simulink model "eurofusion_force_control"  (R2025b)
settings: Solver=ode1  StartTime=0.0  StopTime=100  FixedStep=dt  RelTol=1e-3
model workspace (MAT data in the model file):
  Kd_orient_value = 10
  Kd_pos_value = 100
  Kf_pos = 1
  Kf_rot = 1
  Kp_orient_value = 1
  Kp_pos_value = 1
  Md_pos = 1
  Md_rot = 1
  dt = 0.001
libraries: sdu_controllers x5
settings Model: Creator=eld  LastModifiedBy=madla

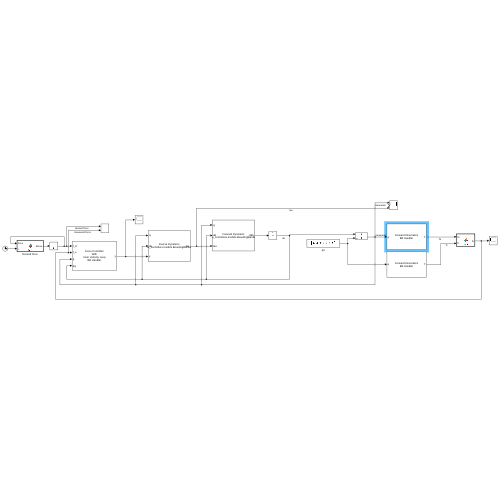
[thumbnail: Simulink's stored preview of the top-level diagram]
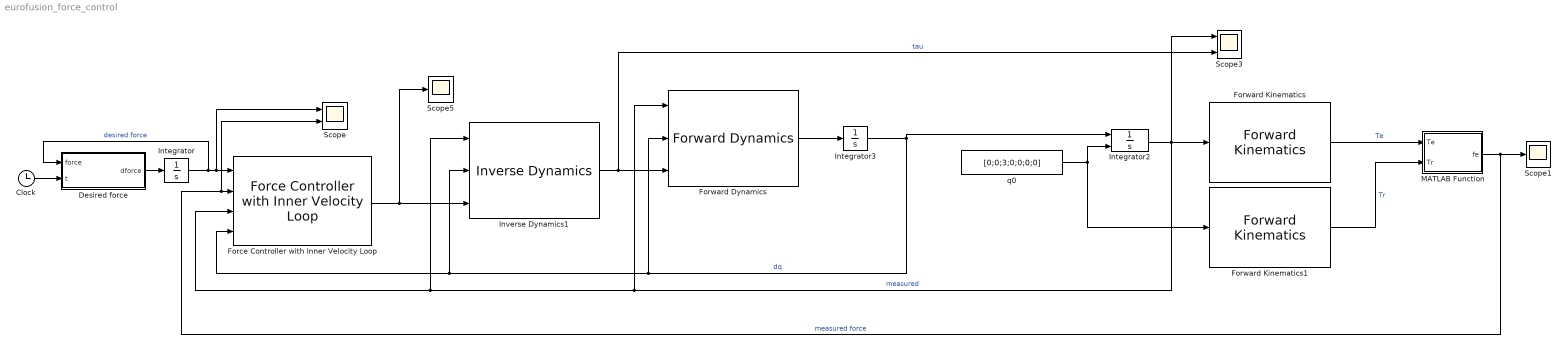
== system eurofusion_force_control ==
  Clock : Clock
  Desired force : MATLAB Function  TreatAsAtomicUnit=on
  Force Controller with Inner Velocity Loop : sdu_controllers/Controllers/Force Controller with Inner Velocity Loop  Kp=diag([ones(1,3)*Kp_pos_value, ones(1,3)*Kp_orient_value])  Kd=diag([ones(1,3)*Kd_pos_value, ones(1,3)*Kd_orient_value])  Md=diag([ones(1,3)*Md_pos, ones(1,3)*Md_rot])  Kf=diag([ones(1,3)*Kf_pos, ones(1,3)*Kf_rot])  RobotType=BB Handler  SimulateUsing=Interpreted execution
      settings: SourceProductName=SDU Controllers
  Forward Dynamics : sdu_controllers/Dynamics/Forward Dynamics  robot_model=bbrobot  SimulateUsing=Interpreted execution
      settings: SourceProductName=SDU Controllers
  Forward Kinematics : sdu_controllers/Kinematics/Forward Kinematics  RobotType=BB Handler  SimulateUsing=Interpreted execution
      settings: SourceProductName=SDU Controllers
  Forward Kinematics1 : sdu_controllers/Kinematics/Forward Kinematics  RobotType=BB Handler  SimulateUsing=Interpreted execution
      settings: SourceProductName=SDU Controllers
  Integrator : Integrator  InitialCondition=zeros(6, 1)
  Integrator2 : Integrator  InitialConditionSource=external  InitialCondition=[0; 0; 3.; 0; 0; 0; 0]
  Integrator3 : Integrator  InitialCondition=zeros(7,1)
  Inverse Dynamics1 : sdu_controllers/Dynamics/Inverse Dynamics  robot_model=bbrobot  SimulateUsing=Interpreted execution
      settings: SourceProductName=SDU Controllers
  MATLAB Function : MATLAB Function  TreatAsAtomicUnit=on
  Scope : Scope  NumInputPorts=2
      settings: ActiveDisplayYMinimum=-124.99686  ActiveDisplayYMaximum=125.00314
  Scope1 : Scope
      settings: ActiveDisplayYMinimum=-124.756  ActiveDisplayYMaximum=124.76228  DataLoggingVariableName=ScopeData2
  Scope3 : Scope  NumInputPorts=3
      settings: ActiveDisplayYMinimum=-395.45944  ActiveDisplayYMaximum=3526.23399  DataLoggingVariableName=ScopeData3
  Scope5 : Scope
      settings: ActiveDisplayYMinimum=-0.01202  ActiveDisplayYMaximum=0.06877  DataLoggingVariableName=ScopeData5
  q0 : Constant  Value=[0;0;3;0;0;0;0]
  wires:
  Inverse Dynamics1/1 -> Forward Dynamics/3, Scope3/3  "tau"
  Force Controller with Inner Velocity Loop/1 -> Scope5/1, Inverse Dynamics1/3
  Integrator2/1 -> Scope3/1, Forward Kinematics/1, Forward Dynamics/1, Force Controller with Inner Velocity Loop/3, Inverse Dynamics1/1  "measured"
  Integrator3/1 -> Integrator2/1, Forward Dynamics/2, Force Controller with Inner Velocity Loop/4, Inverse Dynamics1/2  "dq"
  Forward Dynamics/1 -> Integrator3/1
  Desired force/1(dforce) -> Integrator/1
  Integrator/1 -> Desired force/1(force), Scope/1, Force Controller with Inner Velocity Loop/1  "desired force"
  Clock/1 -> Desired force/2(t)
  q0/1 -> Forward Kinematics1/1, Integrator2/2
  Forward Kinematics/1 -> MATLAB Function/1(Te)  "Te"
  Forward Kinematics1/1 -> MATLAB Function/2(Tr)  "Tr"
  MATLAB Function/1(fe) -> Scope1/1, Scope/2, Force Controller with Inner Velocity Loop/2  "measured force"

== matlab function eurofusion_force_control/Desired force ==
  data: force input; dforce output; t input
function dforce = fcn(force, t)

dforce = [0;
          pi * cos(pi * t / 50) / 5;
          2 * pi * cos(pi * t / 50);
          0;
          0;
          0];

== matlab function eurofusion_force_control/MATLAB Function ==
  data: Te input; fe output; Tr input
function fe = env(Te, Tr)

xe = Te(1:3, 4);
xr = Tr(1:3, 4);

Kenv = 100;
fe = [Kenv * (xe - xr);
      zeros(3, 1)];
